simulink model "lab2zad2"  (R2021a)
settings: Solver=VariableStepAuto  StartTime=0.0  StopTime=61  RelTol=1e-3
libraries: simulink x1
settings Model: Creator=User  LastModifiedBy=pe4en
settings DebuggingCC: UnconnectedInputMsg=none  UnconnectedOutputMsg=none  UnconnectedLineMsg=none
settings ModelReferenceCC: EnableRefExpFcnMdlSchedulingChecks=off
settings RTWCC: Description=Generic Real-Time Target  DLArmComputeVersion=20.02.1

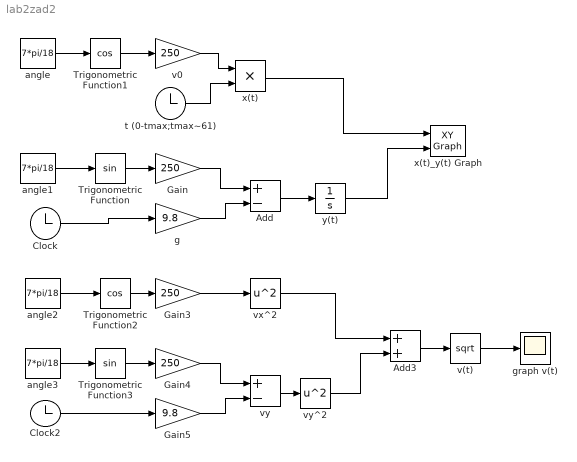
== system lab2zad2 ==
  Add : Sum  Inputs=+-
  Add3 : Sum
  Clock : Clock
  Clock2 : Clock
  Gain : Gain  Gain=250
  Gain3 : Gain  Gain=250
  Gain4 : Gain  Gain=250
  Gain5 : Gain  Gain=9.8
  Trigonometric Function : Trigonometry
  Trigonometric Function1 : Trigonometry  Operator=cos
  Trigonometric Function2 : Trigonometry  Operator=cos
  Trigonometric Function3 : Trigonometry
  angle{,1..3} (4 alike) : Constant  Value=7*pi/18
  g : Gain  Gain=9.8
  graph v(t) : Scope
  t (0-tmax;tmax~61) : Clock
  v(t) : Sqrt  SaturateOnIntegerOverflow=on
  v0 : Gain  Gain=250
  vx^2 : Math  Operator=square  SaturateOnIntegerOverflow=on
  vy : Sum  Inputs=+-
  vy^2 : Math  Operator=square  SaturateOnIntegerOverflow=on
  x(t) : Product  Inputs=**
  x(t)_y(t) Graph : simulink/Sinks/XY Graph  xmin=-1  xmax=1000  ymin=-1  ymax=2000  st=-1
  y(t) : Integrator  UpperSaturationLimit=61  LowerSaturationLimit=0
  wires:
  angle1/1 -> Trigonometric Function/1
  Trigonometric Function/1 -> Gain/1
  Gain/1 -> Add/1
  g/1 -> Add/2
  Clock/1 -> g/1
  Add/1 -> y(t)/1
  Trigonometric Function1/1 -> v0/1
  angle/1 -> Trigonometric Function1/1
  v0/1 -> x(t)/1
  t (0-tmax;tmax~61)/1 -> x(t)/2
  angle2/1 -> Trigonometric Function2/1
  Trigonometric Function2/1 -> Gain3/1
  Gain4/1 -> vy/1
  angle3/1 -> Trigonometric Function3/1
  vy/1 -> vy^2/1
  Trigonometric Function3/1 -> Gain4/1
  Clock2/1 -> Gain5/1
  Gain5/1 -> vy/2
  Gain3/1 -> vx^2/1
  vy^2/1 -> Add3/2
  vx^2/1 -> Add3/1
  Add3/1 -> v(t)/1
  v(t)/1 -> graph v(t)/1
  y(t)/1 -> x(t)_y(t) Graph/2
  x(t)/1 -> x(t)_y(t) Graph/1
